simulink model "bldc_control_sim"  (R2021b)
settings: Solver=VariableStepAuto  StartTime=0.0  StopTime=30  RelTol=1e-3
InitFcn:
  | run bldc_control_params
values from neighbouring files (symbols this model uses):
  B = 2.63687521782e-06    [bldc_control_params.m]
  delay_Currents = 2    [bldc_control_params.m]
  enc_res = 16    [bldc_control_params.m]
  J = 7.06155183-06    (= 1.06155183)    [bldc_control_params.m]
  Ki_i = 3.7e3    (= 3700)    [bldc_control_params.m]
  Ki_speed = 0.1    [bldc_control_params.m]
  Kp_i = 2    [bldc_control_params.m]
  Kp_speed = 5    [bldc_control_params.m]
  poles = 14    [bldc_control_params.m]
  PositionOffset = 0.0    (= 0)    [bldc_control_params.m]
  T_pwm = 20000    [bldc_control_params.m]
  T_rated = 2    [bldc_control_params.m]
  Ts = 5.0e-5    (= 5e-05)    [bldc_control_params.m]
  Ts_inverter = 2.5e-5    (= 2.5e-05)    [bldc_control_params.m]
  Ts_motor = 2.5e-5    (= 2.5e-05)    [bldc_control_params.m]
  Ts_simulink = 2.5e-5    (= 2.5e-05)    [bldc_control_params.m]
  Ts_speed = 5.0e-4    (= 0.0005)    [bldc_control_params.m]
  V_dc = 15    [bldc_control_params.m]
libraries: mcbcontrolslib x19, mcbpositiondecoderlib x4, autolibpmsmexterior x1
settings Model: Creator=vasko  LastModifiedBy=vasko

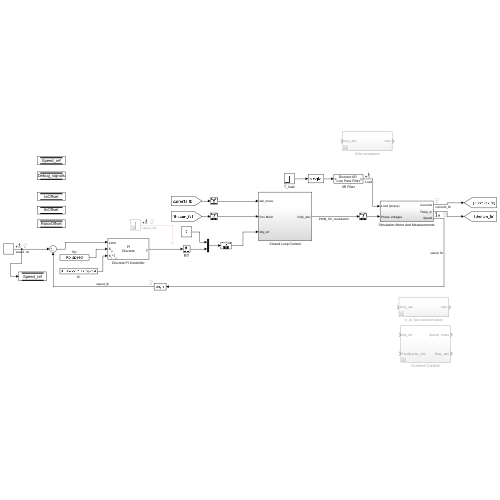
[thumbnail: Simulink's stored preview of the top-level diagram]
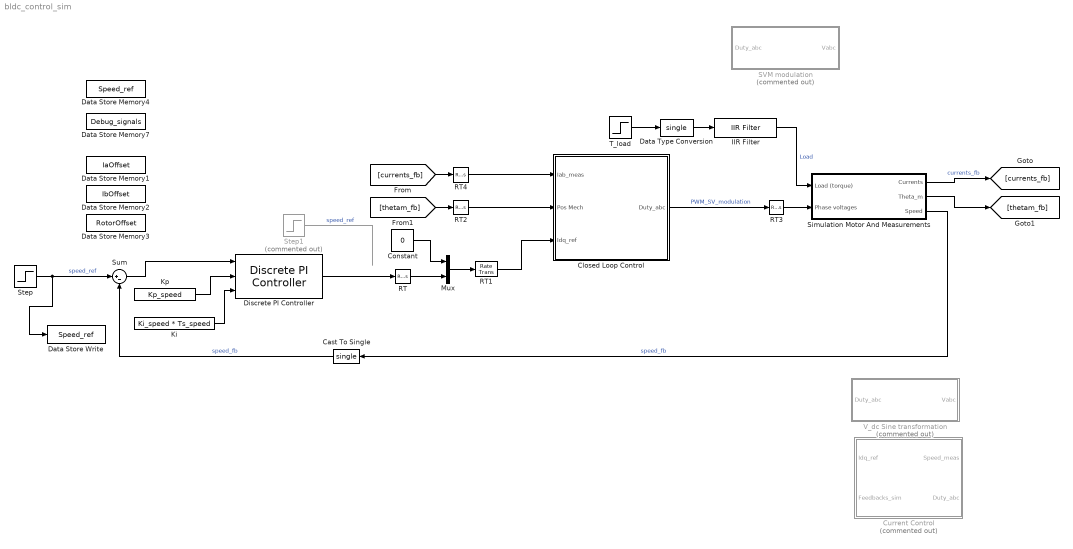
== system bldc_control_sim ==
  Cast To Single : DataTypeConversion  OutDataTypeStr=single
  Closed Loop Control : Subsystem
  Constant : Constant  Value=0  OutDataTypeStr=single
  Current Control : Subsystem  Commented=on
      settings: RTWSystemCode=Nonreusable function
  Data Store Memory1 : DataStoreMemory  DataStoreName=IaOffset  InitialValue=2064  ShowAdditionalParam=off  OutDataTypeStr=uint16
  Data Store Memory2 : DataStoreMemory  DataStoreName=IbOffset  InitialValue=2064  ShowAdditionalParam=off  OutDataTypeStr=uint16
  Data Store Memory3 : DataStoreMemory  DataStoreName=RotorOffset  InitialValue=2064  ShowAdditionalParam=off  OutDataTypeStr=uint16
  Data Store Memory4 : DataStoreMemory  DataStoreName=Speed_ref  ShowAdditionalParam=off  OutDataTypeStr=dataType
  Data Store Memory7 : DataStoreMemory  DataStoreName=Debug_signals  InitialValue=5  ShowAdditionalParam=off  OutDataTypeStr=uint16
  Data Store Write : DataStoreWrite  DataStoreName=Speed_ref  IndexOptions=Index vector (dialog)  Indices=1  OutputSizes=1
  Data Type Conversion : DataTypeConversion  OutDataTypeStr=single
  Discrete PI Controller : mcbcontrolslib/Discrete PI Controller
      settings: SourceProductBaseCode=MT
  IIR Filter : mcbcontrolslib/IIR Filter  VariantControl=Low Pass Filter  VariantSelect=Low-pass  Filter_constant=0.01  advancedSettings=off  Ts=50e-6  cutOff_freq=32.1525
      settings: SourceProductBaseCode=MT
  Ki : Constant  Value=Ki_speed * Ts_speed  OutDataTypeStr=dataType  SampleTime=-1
  Kp : Constant  Value=Kp_speed  OutDataTypeStr=dataType  SampleTime=-1
  Mux : Mux  Inputs=2
  RT : RateTransition  Deterministic=off  OutPortSampleTime=Ts_speed
  RT{1..4} (4 alike) : RateTransition  Deterministic=off
  SVM modulation : Subsystem  Commented=on
  Simulation Motor And Measurements : Subsystem
  Step : Step  After=2  OutDataTypeStr=single  SampleTime=Ts_simulink
  Step1 : Step  Commented=on  After=100  OutDataTypeStr=single  SampleTime=Ts_simulink
  Sum : Sum  Inputs=|+-
  T_load : Step  Time=1.5  After=0*T_rated  SampleTime=Ts_simulink
  V_dc Sine transformation : Subsystem  Commented=on
  wires:
  Simulation Motor And Measurements/1(Currents) -> [currents_fb]  "currents_fb"
  [currents_fb] -> RT4/1
  Step/1 -> Sum/1, Data Store Write/1  "speed_ref"
  RT/1 -> Mux/2
  Data Type Conversion/1 -> IIR Filter/1
  IIR Filter/1 -> Simulation Motor And Measurements/1(Load (torque))  "Load"
  Constant/1 -> Mux/1
  Mux/1 -> RT1/1
  T_load/1 -> Data Type Conversion/1
  Closed Loop Control/1(Duty_abc) -> RT3/1  "PWM_SV_modulation"
  RT2/1 -> Closed Loop Control/2(Pos Mech)
  RT4/1 -> Closed Loop Control/1(Iab_meas)
  RT1/1 -> Closed Loop Control/3(Idq_ref)
  RT3/1 -> Simulation Motor And Measurements/2(Phase voltages)
  [thetam_fb] -> RT2/1
  Simulation Motor And Measurements/2(Theta_m) -> [thetam_fb]
  Simulation Motor And Measurements/3(Speed) -> Cast To Single/1  "speed_fb"
  Sum/1 -> Discrete PI Controller/1
  Ki/1 -> Discrete PI Controller/3
  Kp/1 -> Discrete PI Controller/2
  Cast To Single/1 -> Sum/2  "speed_fb"
  Step1/1 -> ?  "speed_ref"
  Discrete PI Controller/1 -> RT/1

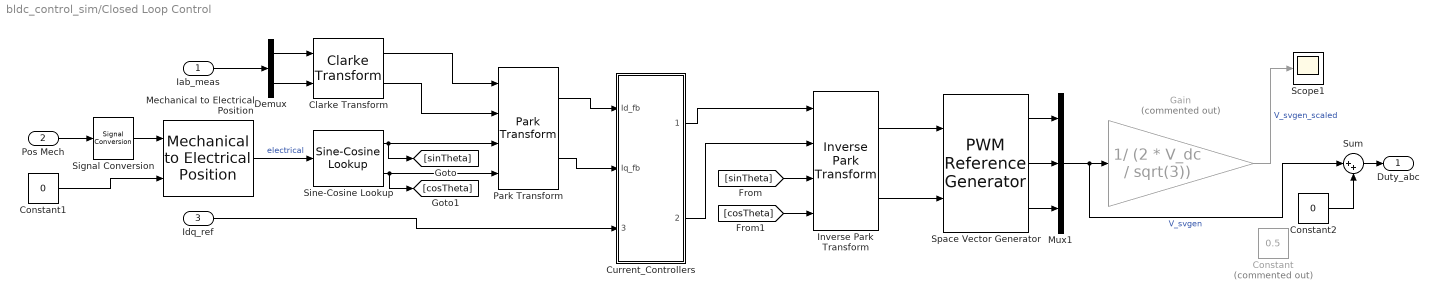
== system bldc_control_sim/Closed Loop Control ==
  Iab_meas : Inport
  Pos Mech : Inport  Port=2
  Idq_ref : Inport  Port=3
  Clarke Transform : mcbcontrolslib/Clarke Transform  VariantControl=Variant2
  Constant : Constant  Commented=on  Value=0.5  OutDataTypeStr=dataType  SampleTime=-1
  Constant1 : Constant  Value=0
  Constant2 : Constant  Value=0
  Current_Controllers : Subsystem
  Demux : Demux  Outputs=2
  Gain : Gain  Commented=on  Gain=1/ (2 * V_dc / sqrt(3))  RndMeth=Simplest  OutDataTypeStr=Inherit: Same as input
  Inverse Park Transform : mcbcontrolslib/Inverse Park Transform  AxisAlignment=D-axis
  Mechanical to Electrical Position : mcbpositiondecoderlib/Mechanical to Electrical Position  NrPP=poles  selectedRange=Radians  MechOfstInputType=Input port  mechOffsetIn=0  maxAngleIn=2*pi  InputDataType=dataType  VariantSelect=floating-point
      settings: SourceProductBaseCode=MT
  Mux1 : Mux  Inputs=3
  Park Transform : mcbcontrolslib/Park Transform  AxisAlignment=D-axis
      settings: SourceProductBaseCode=MT
  Scope1 : Scope
  Signal Conversion : SignalConversion  OverrideOpt=off
  Sine-Cosine Lookup : mcbcontrolslib/Sine-Cosine Lookup  AngleInput=Radians  N_points=1024
      settings: SourceProductBaseCode=MT
  Space Vector Generator : mcbcontrolslib/PWM Reference Generator  inSignal=Valphabeta  modType=SVM: space vector modulation
      settings: SourceProductBaseCode=MT
  Sum : Sum  Inputs=|++
  Duty_abc : Outport  VectorParamsAs1DForOutWhenUnconnected=off
  wires:
  Iab_meas/1 -> Demux/1
  Park Transform/2 -> Current_Controllers/2(Iq_fb)
  Park Transform/1 -> Current_Controllers/1(Id_fb)
  Sine-Cosine Lookup/2 -> Park Transform/4, [cosTheta]
  Clarke Transform/1 -> Park Transform/1
  Idq_ref/1 -> Current_Controllers/3(Idq_ref)
  Sine-Cosine Lookup/1 -> [sinTheta], Park Transform/3
  Clarke Transform/2 -> Park Transform/2
  [cosTheta] -> Inverse Park Transform/4
  Demux/2 -> Clarke Transform/2
  Demux/1 -> Clarke Transform/1
  [sinTheta] -> Inverse Park Transform/3
  Current_Controllers/1(Vd_ref) -> Inverse Park Transform/1
  Current_Controllers/2(Vq_ref) -> Inverse Park Transform/2
  Inverse Park Transform/2 -> Space Vector Generator/2
  Mux1/1 -> Sum/1, Gain/1  "V_svgen"
  Space Vector Generator/1 -> Mux1/1
  Gain/1 -> Scope1/1  "V_svgen_scaled"
  Inverse Park Transform/1 -> Space Vector Generator/1
  Space Vector Generator/2 -> Mux1/2
  Space Vector Generator/3 -> Mux1/3
  Sum/1 -> Duty_abc/1
  Pos Mech/1 -> Signal Conversion/1
  Mechanical to Electrical Position/1 -> Sine-Cosine Lookup/1  "electrical"
  Constant1/1 -> Mechanical to Electrical Position/2
  Constant2/1 -> Sum/2
  Signal Conversion/1 -> Mechanical to Electrical Position/1

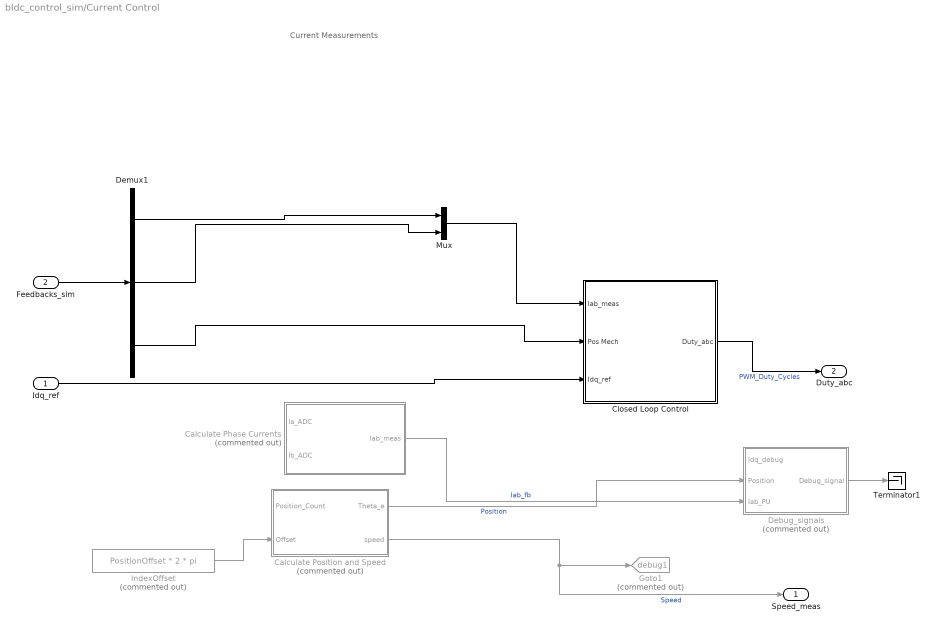
== system bldc_control_sim/Current Control ==
  note: Current Measurements
  Idq_ref : Inport
  Feedbacks_sim : Inport  Port=2
  " Calculate Position and Speed" : Subsystem  Commented=on
  Calculate Phase Currents : Subsystem  Commented=on
  Closed Loop Control : Subsystem
  Debug_signals : Subsystem  Commented=on
  Demux1 : Demux  Outputs=3
  Goto1 : Goto  Commented=on  GotoTag=debug1  TagVisibility=global
  IndexOffset : Constant  Commented=on  Value=PositionOffset * 2 * pi  OutDataTypeStr=dataType  SampleTime=-1
  Mux : Mux  Inputs=2
  Terminator1 : Terminator
  Speed_meas : Outport  InitialOutput=0  VectorParamsAs1DForOutWhenUnconnected=off
  Duty_abc : Outport  Port=2  VectorParamsAs1DForOutWhenUnconnected=off
  wires:
  " Calculate Position and Speed"/1(Theta_e) -> Debug_signals/2(Position)  "Position"
  " Calculate Position and Speed"/2(speed) -> Speed_meas/1, Goto1/1  "Speed"
  Calculate Phase Currents/1(Iab_meas) -> Debug_signals/3(Iab_PU)  "Iab_fb"
  Debug_signals/1(Debug_signal) -> Terminator1/1
  IndexOffset/1 -> " Calculate Position and Speed"/2(Offset)
  Idq_ref/1 -> Closed Loop Control/3(Idq_ref)
  Closed Loop Control/1(Duty_abc) -> Duty_abc/1  "PWM_Duty_Cycles"
  Feedbacks_sim/1 -> Demux1/1
  Demux1/1 -> Mux/1
  Demux1/2 -> Mux/2
  Demux1/3 -> Closed Loop Control/2(Pos Mech)
  Mux/1 -> Closed Loop Control/1(Iab_meas)

== system bldc_control_sim/SVM modulation ==
  Duty_abc : Inport
  Average_Value_Inverter : Subsystem
  Constant2 : Constant  Value=V_dc  OutDataTypeStr=single  SampleTime=-1
  Data Type Conversion1 : DataTypeConversion  OutDataTypeStr=single  RndMeth=Simplest
  Demux : Demux  Outputs=3
  Inverter_delay : DiscreteTransferFcn  Numerator=[1-exp(-Ts_inverter/(T_pwm/2))]  Denominator=[1 -exp(-Ts_inverter/(T_pwm/2))]  RndMeth=Simplest
  Mux : Mux  Inputs=3
  Rate Transition3 : RateTransition  Integrity=off  OutPortSampleTime=Ts_inverter
  Vabc : Outport  VectorParamsAs1DForOutWhenUnconnected=off
  wires:
  Average_Value_Inverter/2(Vb) -> Mux/2
  Mux/1 -> Inverter_delay/1
  Constant2/1 -> Average_Value_Inverter/4(Vdc)
  Average_Value_Inverter/3(Vc) -> Mux/3
  Average_Value_Inverter/1(Va) -> Mux/1
  Demux/1 -> Average_Value_Inverter/1(Vao)
  Demux/3 -> Average_Value_Inverter/3(Vco)
  Demux/2 -> Average_Value_Inverter/2(Vbo)
  Data Type Conversion1/1 -> Rate Transition3/1
  Rate Transition3/1 -> Demux/1
  Inverter_delay/1 -> Vabc/1
  Duty_abc/1 -> Data Type Conversion1/1

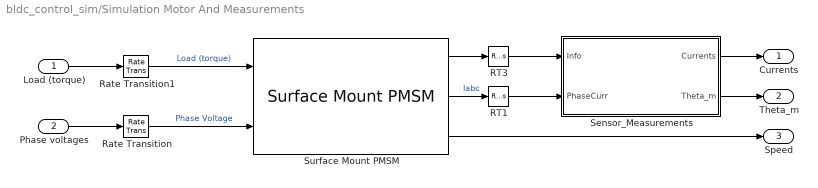
== system bldc_control_sim/Simulation Motor And Measurements ==
  Load (torque) : Inport
  Phase voltages : Inport  Port=2
  RT1 : RateTransition  Deterministic=off  OutPortSampleTime=Ts_simulink
  RT3 : RateTransition  Deterministic=off  OutPortSampleTime=Ts_simulink
  Rate Transition : RateTransition  Integrity=off  OutPortSampleTime=Ts_motor
  Rate Transition1 : RateTransition  Integrity=off  OutPortSampleTime=Ts_motor
  Sensor_Measurements : Subsystem
  Surface Mount PMSM : autolibpmsmexterior/Surface Mount PMSM  port_config=Torque  sim_type=Discrete  Ts=Ts_motor  P=poles  Rs=Rs  Ldq_=Ld  KConstText=Permanent flux linkage constant (lambda_pm):  lambda_pm=FluxPM  Ke=159.9771  Kt=1.323  mechanical=[J, B, 0]  idq0=[0 0]  theta_init=0  omega_init=0  KConst=FluxPM  lambda_pm_calc=FluxPM  RefBlkName='autolibpmsmexterior/Surface Mount PMSM'  aMode=5  Ldq="[0.00105     0.00105]"
      settings: SourceProductBaseCode=PW,DR,MT,UV,VE
  Currents : Outport  VectorParamsAs1DForOutWhenUnconnected=off
  Theta_m : Outport  Port=2  VectorParamsAs1DForOutWhenUnconnected=off
  Speed : Outport  Port=3  VectorParamsAs1DForOutWhenUnconnected=off
  wires:
  Rate Transition1/1 -> Surface Mount PMSM/1  "Load (torque)"
  Surface Mount PMSM/2 -> RT1/1  "Iabc"
  Surface Mount PMSM/3 -> Speed/1
  Rate Transition/1 -> Surface Mount PMSM/2  "Phase Voltage"
  RT1/1 -> Sensor_Measurements/2(PhaseCurr)
  Phase voltages/1 -> Rate Transition/1
  RT3/1 -> Sensor_Measurements/1(Info)
  Surface Mount PMSM/1 -> RT3/1
  Load (torque)/1 -> Rate Transition1/1
  Sensor_Measurements/1(Currents) -> Currents/1
  Sensor_Measurements/2(Theta_m) -> Theta_m/1

== system bldc_control_sim/V_dc Sine transformation ==
  Duty_abc : Inport
  Average_Value_Inverter : Subsystem
  Constant2 : Constant  Value=V_dc  OutDataTypeStr=single  SampleTime=-1
  Data Type Conversion1 : DataTypeConversion  OutDataTypeStr=single  RndMeth=Simplest
  Demux : Demux  Outputs=3
  Mux : Mux  Inputs=3
  Rate Transition3 : RateTransition  Integrity=off  OutPortSampleTime=Ts_inverter
  Vabc : Outport  VectorParamsAs1DForOutWhenUnconnected=off
  wires:
  Average_Value_Inverter/2(Vb) -> Mux/2
  Constant2/1 -> Average_Value_Inverter/4(Vdc)
  Average_Value_Inverter/3(Vc) -> Mux/3
  Average_Value_Inverter/1(Va) -> Mux/1
  Demux/1 -> Average_Value_Inverter/1(Vao)
  Demux/3 -> Average_Value_Inverter/3(Vco)
  Demux/2 -> Average_Value_Inverter/2(Vbo)
  Data Type Conversion1/1 -> Rate Transition3/1
  Rate Transition3/1 -> Demux/1
  Mux/1 -> Vabc/1  "V_inv_abc"
  Duty_abc/1 -> Data Type Conversion1/1

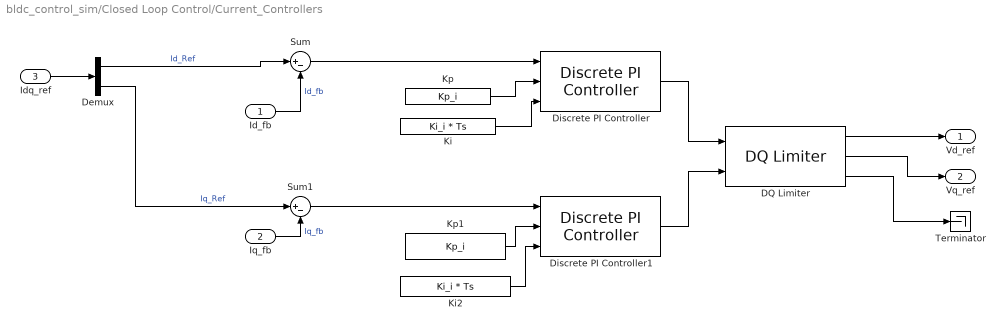
== system bldc_control_sim/Closed Loop Control/Current_Controllers ==
  Id_fb : Inport
  Iq_fb : Inport  Port=2
  Idq_ref : Inport  Port=3
  DQ Limiter : mcbcontrolslib/DQ Limiter  Vmax=Idq_lim
      settings: SourceProductBaseCode=MT
  Demux : Demux  Outputs=2
  Discrete PI Controller : mcbcontrolslib/Discrete PI Controller
      settings: SourceProductBaseCode=MT
  Discrete PI Controller1 : mcbcontrolslib/Discrete PI Controller
      settings: SourceProductBaseCode=MT
  Ki : Constant  Value=Ki_i * Ts  OutDataTypeStr=dataType  SampleTime=-1
  Ki2 : Constant  Value=Ki_i * Ts  OutDataTypeStr=dataType  SampleTime=-1
  Kp : Constant  Value=Kp_i  OutDataTypeStr=dataType  SampleTime=-1
  Kp1 : Constant  Value=Kp_i  OutDataTypeStr=dataType  SampleTime=-1
  Sum : Sum  Inputs=|+-  OutDataTypeStr=Inherit: Same as first input
  Sum1 : Sum  Inputs=|+-  OutDataTypeStr=Inherit: Same as first input
  Terminator : Terminator
  Vd_ref : Outport  VectorParamsAs1DForOutWhenUnconnected=off
  Vq_ref : Outport  Port=2  VectorParamsAs1DForOutWhenUnconnected=off
  wires:
  Iq_fb/1 -> Sum1/2  "Iq_fb"
  Id_fb/1 -> Sum/2  "Id_fb"
  Demux/1 -> Sum/1  "Id_Ref"
  Demux/2 -> Sum1/1  "Iq_Ref"
  Idq_ref/1 -> Demux/1
  DQ Limiter/2 -> Vq_ref/1
  DQ Limiter/1 -> Vd_ref/1
  DQ Limiter/3 -> Terminator/1
  Ki/1 -> Discrete PI Controller/3
  Sum/1 -> Discrete PI Controller/1
  Kp/1 -> Discrete PI Controller/2
  Sum1/1 -> Discrete PI Controller1/1
  Ki2/1 -> Discrete PI Controller1/3
  Kp1/1 -> Discrete PI Controller1/2
  Discrete PI Controller/1 -> DQ Limiter/1
  Discrete PI Controller1/1 -> DQ Limiter/2

== system bldc_control_sim/Current Control/ Calculate Position and Speed ==
  Position_Count : Inport
  Offset : Inport  Port=2
  Cast To Single : DataTypeConversion  OutDataTypeStr=single
  Gain : Gain  Gain=2*pi/(2^enc_res)
  IIR Filter : mcbcontrolslib/IIR Filter  VariantControl=Low Pass Filter  VariantSelect=Low-pass  Filter_constant=0.01  advancedSettings=off  Ts=50e-6  cutOff_freq=32.1525
      settings: SourceProductBaseCode=MT
  Mechanical to Electrical Position : mcbpositiondecoderlib/Mechanical to Electrical Position  NrPP=poles  selectedRange=Radians  MechOfstInputType=Input port  mechOffsetIn=0  maxAngleIn=2*pi  InputDataType=dataType  VariantSelect=floating-point
      settings: SourceProductBaseCode=MT
  Speed Measurement : mcbpositiondecoderlib/Speed Measurement  PositionUnit=Radians  PositionScalingDatatype=uint32  SpeedCalculationMode=Time interval for speed calculation  SampleTimeAsync=Ts  MaximumApplicationSpeed=6000  SpeedResolution=5e-6  DelayLength=20  MaximumMeasurableSpeed=29999  MeasurableSpeedResolution=1.397e-05  SpeedUnit=Radians/Sec  PerUnitSpeed=PU_System.N_base  SpeedDataType=dataType
      settings: SourceProductBaseCode=MT
  Theta_e : Outport  VectorParamsAs1DForOutWhenUnconnected=off
  speed : Outport  Port=2  VectorParamsAs1DForOutWhenUnconnected=off
  wires:
  Speed Measurement/1 -> IIR Filter/1
  Mechanical to Electrical Position/1 -> Theta_e/1
  Position_Count/1 -> Gain/1
  Offset/1 -> Mechanical to Electrical Position/2
  IIR Filter/1 -> speed/1
  Gain/1 -> Cast To Single/1
  Cast To Single/1 -> Speed Measurement/1, Mechanical to Electrical Position/1  "angle"

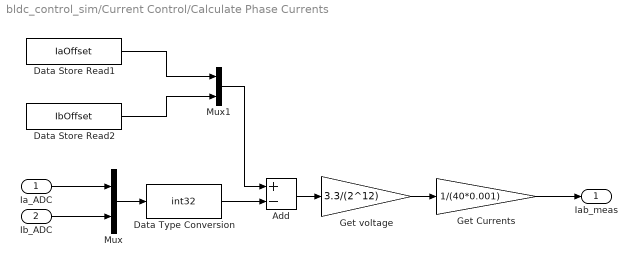
== system bldc_control_sim/Current Control/Calculate Phase Currents ==
  Ia_ADC : Inport
  Ib_ADC : Inport  Port=2
  Add : Sum  Inputs=+-
  Data Store Read1 : DataStoreRead  DataStoreName=IaOffset  IndexOptions=Index vector (dialog)  Indices=1  OutputSizes=1
  Data Store Read2 : DataStoreRead  DataStoreName=IbOffset  IndexOptions=Index vector (dialog)  Indices=1  OutputSizes=1
  Data Type Conversion : DataTypeConversion  OutDataTypeStr=int32  ConvertRealWorld=Stored Integer (SI)  RndMeth=Simplest
  Get Currents : Gain  Gain=1/(40*0.001)  OutDataTypeStr=dataType  RndMeth=Simplest
  Get voltage : Gain  Gain=3.3/(2^12)
  Mux : Mux  Inputs=2
  Mux1 : Mux  Inputs=2
  Iab_meas : Outport  VectorParamsAs1DForOutWhenUnconnected=off
  wires:
  Data Type Conversion/1 -> Add/2
  Ia_ADC/1 -> Mux/1
  Ib_ADC/1 -> Mux/2
  Mux/1 -> Data Type Conversion/1
  Data Store Read1/1 -> Mux1/1
  Data Store Read2/1 -> Mux1/2
  Mux1/1 -> Add/1
  Get Currents/1 -> Iab_meas/1
  Add/1 -> Get voltage/1
  Get voltage/1 -> Get Currents/1

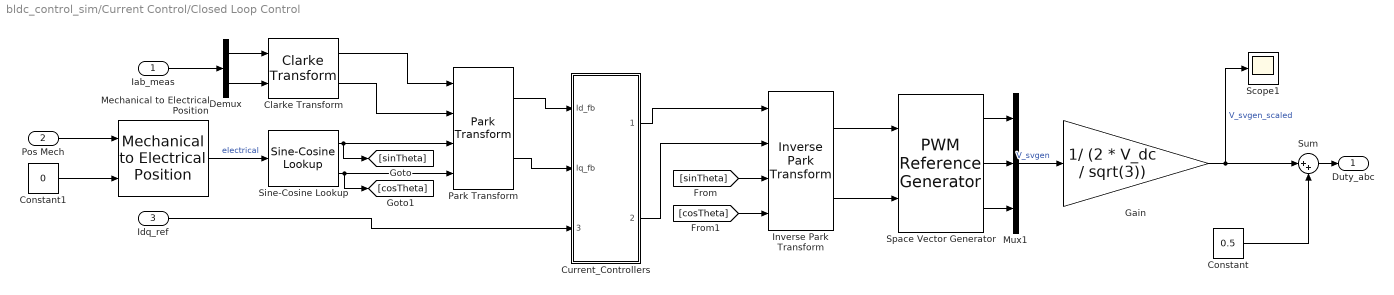
== system bldc_control_sim/Current Control/Closed Loop Control ==
  Iab_meas : Inport
  Pos Mech : Inport  Port=2
  Idq_ref : Inport  Port=3
  Clarke Transform : mcbcontrolslib/Clarke Transform  VariantControl=Variant2
  Constant : Constant  Value=0.5  OutDataTypeStr=dataType  SampleTime=-1
  Constant1 : Constant  Value=0
  Current_Controllers : Subsystem
  Demux : Demux  Outputs=2
  Gain : Gain  Gain=1/ (2 * V_dc / sqrt(3))  RndMeth=Simplest  OutDataTypeStr=Inherit: Same as input
  Inverse Park Transform : mcbcontrolslib/Inverse Park Transform  AxisAlignment=D-axis
  Mechanical to Electrical Position : mcbpositiondecoderlib/Mechanical to Electrical Position  NrPP=poles  selectedRange=Radians  MechOfstInputType=Input port  mechOffsetIn=0  maxAngleIn=2*pi  InputDataType=dataType  VariantSelect=floating-point
      settings: SourceProductBaseCode=MT
  Mux1 : Mux  Inputs=3
  Park Transform : mcbcontrolslib/Park Transform  AxisAlignment=D-axis
      settings: SourceProductBaseCode=MT
  Scope1 : Scope
  Sine-Cosine Lookup : mcbcontrolslib/Sine-Cosine Lookup  AngleInput=Radians  N_points=1024
      settings: SourceProductBaseCode=MT
  Space Vector Generator : mcbcontrolslib/PWM Reference Generator  inSignal=Valphabeta  modType=SVM: space vector modulation
      settings: SourceProductBaseCode=MT
  Sum : Sum  Inputs=|++
  Duty_abc : Outport  VectorParamsAs1DForOutWhenUnconnected=off
  wires:
  Iab_meas/1 -> Demux/1
  Park Transform/2 -> Current_Controllers/2(Iq_fb)
  Park Transform/1 -> Current_Controllers/1(Id_fb)
  Sine-Cosine Lookup/2 -> Park Transform/4, [cosTheta]
  Clarke Transform/1 -> Park Transform/1
  Idq_ref/1 -> Current_Controllers/3(Idq_ref)
  Sine-Cosine Lookup/1 -> [sinTheta], Park Transform/3
  Clarke Transform/2 -> Park Transform/2
  [cosTheta] -> Inverse Park Transform/4
  Demux/2 -> Clarke Transform/2
  Demux/1 -> Clarke Transform/1
  [sinTheta] -> Inverse Park Transform/3
  Current_Controllers/1(Vd_ref) -> Inverse Park Transform/1
  Current_Controllers/2(Vq_ref) -> Inverse Park Transform/2
  Inverse Park Transform/2 -> Space Vector Generator/2
  Constant/1 -> Sum/2
  Mux1/1 -> Gain/1  "V_svgen"
  Space Vector Generator/1 -> Mux1/1
  Gain/1 -> Scope1/1, Sum/1  "V_svgen_scaled"
  Inverse Park Transform/1 -> Space Vector Generator/1
  Space Vector Generator/2 -> Mux1/2
  Space Vector Generator/3 -> Mux1/3
  Sum/1 -> Duty_abc/1
  Pos Mech/1 -> Mechanical to Electrical Position/1
  Mechanical to Electrical Position/1 -> Sine-Cosine Lookup/1  "electrical"
  Constant1/1 -> Mechanical to Electrical Position/2

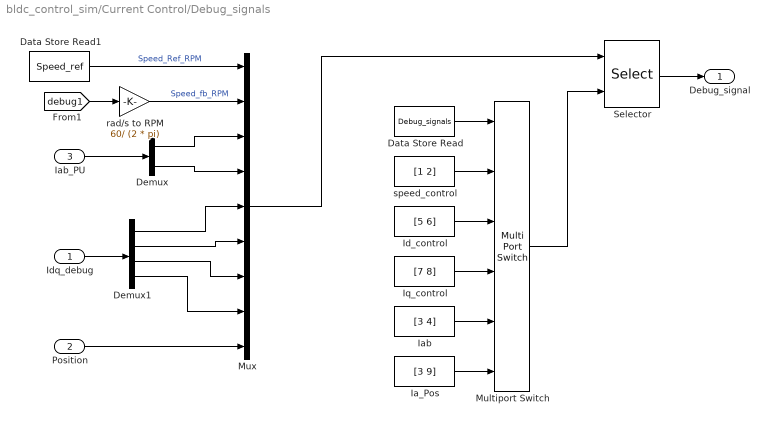
== system bldc_control_sim/Current Control/Debug_signals ==
  Idq_debug : Inport
  Position : Inport  Port=2
  Iab_PU : Inport  Port=3
  Data Store Read : DataStoreRead  DataStoreName=Debug_signals  IndexOptions=Index vector (dialog)  Indices=1  OutputSizes=1
  Data Store Read1 : DataStoreRead  DataStoreName=Speed_ref  IndexOptions=Index vector (dialog)  Indices=1  OutputSizes=1
  Demux : Demux  Outputs=2
  Demux1 : Demux
  Ia_Pos : Constant  Value=[3 9]  OutDataTypeStr=uint16  SampleTime=-1
  Iab : Constant  Value=[3 4]  OutDataTypeStr=uint16  SampleTime=-1
  Id_control : Constant  Value=[5 6]  OutDataTypeStr=uint16  SampleTime=-1
  Iq_control : Constant  Value=[7 8]  OutDataTypeStr=uint16  SampleTime=-1
  Multiport Switch : MultiPortSwitch  Inputs=5  DiagnosticForDefault=Warning  OutDataTypeStr=uint16  RndMeth=Simplest
  Mux : Mux  Inputs=9
  Selector : Selector  InputPortWidth=9  IndexOptions=Index vector (port)  Indices=[1 3]  OutputSizes=1
  rad/s to RPM : Gain  Gain=60/ (2 * pi)  RndMeth=Simplest  OutDataTypeStr=Inherit: Same as input
  speed_control : Constant  Value=[1 2]  OutDataTypeStr=uint16  SampleTime=-1
  Debug_signal : Outport
  wires:
  speed_control/1 -> Multiport Switch/2
  Id_control/1 -> Multiport Switch/3
  Iq_control/1 -> Multiport Switch/4
  Iab/1 -> Multiport Switch/5
  Ia_Pos/1 -> Multiport Switch/6
  Multiport Switch/1 -> Selector/2
  Data Store Read/1 -> Multiport Switch/1
  Selector/1 -> Debug_signal/1
  Iab_PU/1 -> Demux/1
  Demux/1 -> Mux/3
  Demux/2 -> Mux/4
  Demux1/1 -> Mux/5
  Demux1/2 -> Mux/6
  Demux1/3 -> Mux/7
  Demux1/4 -> Mux/8
  Idq_debug/1 -> Demux1/1
  Mux/1 -> Selector/1
  Position/1 -> Mux/9
  [debug1] -> rad/s to RPM/1
  Data Store Read1/1 -> Mux/1  "Speed_Ref_RPM"
  rad/s to RPM/1 -> Mux/2  "Speed_fb_RPM"

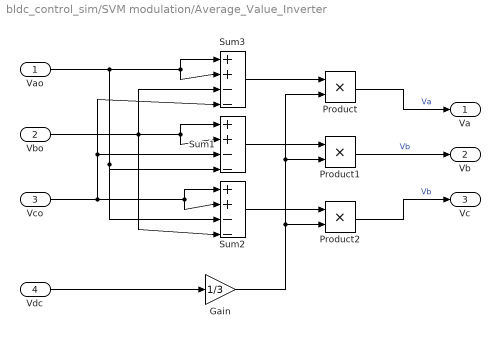
== system bldc_control_sim/SVM modulation/Average_Value_Inverter ==
  Vao : Inport
  Vbo : Inport  Port=2
  Vco : Inport  Port=3
  Vdc : Inport  Port=4
  Gain : Gain  Gain=1/3  RndMeth=Simplest  OutDataTypeStr=Inherit: Same as input
  Product : Product  RndMeth=Simplest  OutDataTypeStr=Inherit: Same as first input
  Product1 : Product  RndMeth=Simplest  OutDataTypeStr=Inherit: Same as first input
  Product2 : Product  RndMeth=Simplest  OutDataTypeStr=Inherit: Same as first input
  Sum1 : Sum  Inputs=|++--  RndMeth=Simplest  OutDataTypeStr=Inherit: Same as first input
  Sum2 : Sum  Inputs=|++--  RndMeth=Simplest  OutDataTypeStr=Inherit: Same as first input
  Sum3 : Sum  Inputs=|++--  RndMeth=Simplest  OutDataTypeStr=Inherit: Same as first input
  Va : Outport  VectorParamsAs1DForOutWhenUnconnected=off
  Vb : Outport  Port=2  VectorParamsAs1DForOutWhenUnconnected=off
  Vc : Outport  Port=3  VectorParamsAs1DForOutWhenUnconnected=off
  wires:
  Product1/1 -> Vb/1  "Vb"
  Gain/1 -> Product/2, Product1/2, Product2/2
  Sum2/1 -> Product2/1
  Vao/1 -> Sum3/1, Sum3/2, Sum1/4, Sum2/3
  Product2/1 -> Vc/1  "Vb"
  Sum1/1 -> Product1/1
  Vdc/1 -> Gain/1
  Sum3/1 -> Product/1
  Product/1 -> Va/1  "Va"
  Vco/1 -> Sum3/4, Sum1/3, Sum2/2, Sum2/1
  Vbo/1 -> Sum1/1, Sum1/2, Sum3/3, Sum2/4

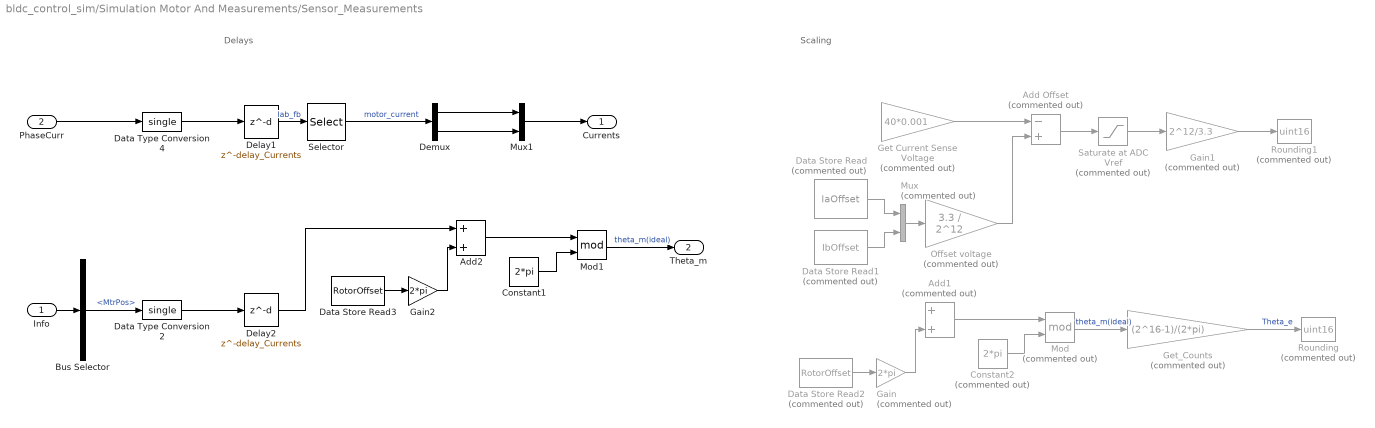
== system bldc_control_sim/Simulation Motor And Measurements/Sensor_Measurements ==
  note: Scaling
  note: Delays
  Info : Inport
  PhaseCurr : Inport  Port=2
  Add Offset : Sum  Commented=on  Inputs=-+  RndMeth=Simplest
  Add1 : Sum  Commented=on  RndMeth=Simplest
  Add2 : Sum  RndMeth=Simplest
  Bus Selector : BusSelector  OutputSignals=MtrPos
  Constant1 : Constant  Value=2*pi  OutDataTypeStr=single  SampleTime=-1
  Constant2 : Constant  Commented=on  Value=2*pi  OutDataTypeStr=single  SampleTime=-1
  Data Store Read : DataStoreRead  Commented=on  DataStoreName=IaOffset  IndexOptions=Index vector (dialog)  Indices=1  OutputSizes=1
  Data Store Read1 : DataStoreRead  Commented=on  DataStoreName=IbOffset  IndexOptions=Index vector (dialog)  Indices=1  OutputSizes=1
  Data Store Read2 : DataStoreRead  Commented=on  DataStoreName=RotorOffset  IndexOptions=Index vector (dialog)  Indices=1  OutputSizes=1
  Data Store Read3 : DataStoreRead  DataStoreName=RotorOffset  IndexOptions=Index vector (dialog)  Indices=1  OutputSizes=1
  Data Type Conversion2 : DataTypeConversion  OutDataTypeStr=single  RndMeth=Simplest
  Data Type Conversion4 : DataTypeConversion  OutDataTypeStr=single  RndMeth=Simplest
  Delay1 : Delay  DelayLength=delay_Currents
  Delay2 : Delay  DelayLength=delay_Currents
  Demux : Demux  Outputs=2
  Gain : Gain  Commented=on  Gain=2*pi
  Gain1 : Gain  Commented=on  Gain=2^12/3.3
  Gain2 : Gain  Gain=2*pi
  Get Current Sense Voltage : Gain  Commented=on  Gain=40*0.001  RndMeth=Simplest  OutDataTypeStr=Inherit: Same as input
  Get_Counts : Gain  Commented=on  Gain=(2^16-1)/(2*pi)  OutDataTypeStr=uint16  RndMeth=Simplest
  Mod : Math  Commented=on  Operator=mod  SaturateOnIntegerOverflow=on
  Mod1 : Math  Operator=mod  SaturateOnIntegerOverflow=on
  Mux : Mux  Commented=on  Inputs=2
  Mux1 : Mux  Inputs=2
  Offset voltage : Gain  Commented=on  Gain=3.3 / 2^12  RndMeth=Simplest
  Rounding : DataTypeConversion  Commented=on  OutDataTypeStr=uint16  RndMeth=Simplest
  Rounding1 : DataTypeConversion  Commented=on  OutDataTypeStr=uint16  RndMeth=Simplest
  Saturate at ADC Vref : Saturate  Commented=on  UpperLimit=3.3  LowerLimit=0
  Selector : Selector  InputPortWidth=3  IndexOptions=Index vector (dialog)  Indices=[1 2]  OutputSizes=1
  Currents : Outport  VectorParamsAs1DForOutWhenUnconnected=off
  Theta_m : Outport  Port=2  VectorParamsAs1DForOutWhenUnconnected=off
  wires:
  Delay1/1 -> Selector/1  "Iab_fb"
  Data Type Conversion4/1 -> Delay1/1
  PhaseCurr/1 -> Data Type Conversion4/1
  Info/1 -> Bus Selector/1
  Bus Selector/1 -> Data Type Conversion2/1  "<MtrPos>"
  Data Type Conversion2/1 -> Delay2/1
  Data Store Read2/1 -> Gain/1
  Add1/1 -> Mod/1
  Get_Counts/1 -> Rounding/1  "Theta_e"
  Mod/1 -> Get_Counts/1  "theta_m(ideal)"
  Mux/1 -> Offset voltage/1
  Get Current Sense Voltage/1 -> Add Offset/1
  Saturate at ADC Vref/1 -> Gain1/1
  Add Offset/1 -> Saturate at ADC Vref/1
  Offset voltage/1 -> Add Offset/2
  Gain1/1 -> Rounding1/1
  Data Store Read1/1 -> Mux/2
  Data Store Read/1 -> Mux/1
  Constant2/1 -> Mod/2
  Gain/1 -> Add1/2
  Selector/1 -> Demux/1  "motor_current"
  Gain2/1 -> Add2/2
  Constant1/1 -> Mod1/2
  Add2/1 -> Mod1/1
  Data Store Read3/1 -> Gain2/1
  Mod1/1 -> Theta_m/1  "theta_m(ideal)"
  Delay2/1 -> Add2/1
  Demux/1 -> Mux1/1
  Demux/2 -> Mux1/2
  Mux1/1 -> Currents/1

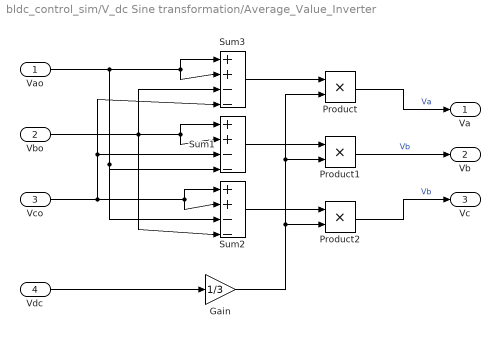
== system bldc_control_sim/V_dc Sine transformation/Average_Value_Inverter ==
  Vao : Inport
  Vbo : Inport  Port=2
  Vco : Inport  Port=3
  Vdc : Inport  Port=4
  Gain : Gain  Gain=1/3  RndMeth=Simplest  OutDataTypeStr=Inherit: Same as input
  Product : Product  RndMeth=Simplest  OutDataTypeStr=Inherit: Same as first input
  Product1 : Product  RndMeth=Simplest  OutDataTypeStr=Inherit: Same as first input
  Product2 : Product  RndMeth=Simplest  OutDataTypeStr=Inherit: Same as first input
  Sum1 : Sum  Inputs=|++--  RndMeth=Simplest  OutDataTypeStr=Inherit: Same as first input
  Sum2 : Sum  Inputs=|++--  RndMeth=Simplest  OutDataTypeStr=Inherit: Same as first input
  Sum3 : Sum  Inputs=|++--  RndMeth=Simplest  OutDataTypeStr=Inherit: Same as first input
  Va : Outport  VectorParamsAs1DForOutWhenUnconnected=off
  Vb : Outport  Port=2  VectorParamsAs1DForOutWhenUnconnected=off
  Vc : Outport  Port=3  VectorParamsAs1DForOutWhenUnconnected=off
  wires:
  Product1/1 -> Vb/1  "Vb"
  Gain/1 -> Product/2, Product1/2, Product2/2
  Sum2/1 -> Product2/1
  Vao/1 -> Sum3/1, Sum3/2, Sum1/4, Sum2/3
  Product2/1 -> Vc/1  "Vb"
  Sum1/1 -> Product1/1
  Vdc/1 -> Gain/1
  Sum3/1 -> Product/1
  Product/1 -> Va/1  "Va"
  Vco/1 -> Sum3/4, Sum1/3, Sum2/2, Sum2/1
  Vbo/1 -> Sum1/1, Sum1/2, Sum3/3, Sum2/4

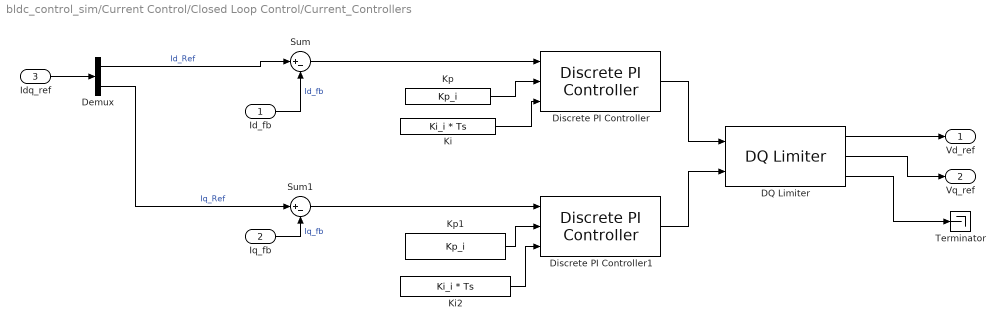
== system bldc_control_sim/Current Control/Closed Loop Control/Current_Controllers ==
  Id_fb : Inport
  Iq_fb : Inport  Port=2
  Idq_ref : Inport  Port=3
  DQ Limiter : mcbcontrolslib/DQ Limiter  Vmax=Idq_lim
      settings: SourceProductBaseCode=MT
  Demux : Demux  Outputs=2
  Discrete PI Controller : mcbcontrolslib/Discrete PI Controller
      settings: SourceProductBaseCode=MT
  Discrete PI Controller1 : mcbcontrolslib/Discrete PI Controller
      settings: SourceProductBaseCode=MT
  Ki : Constant  Value=Ki_i * Ts  OutDataTypeStr=dataType  SampleTime=-1
  Ki2 : Constant  Value=Ki_i * Ts  OutDataTypeStr=dataType  SampleTime=-1
  Kp : Constant  Value=Kp_i  OutDataTypeStr=dataType  SampleTime=-1
  Kp1 : Constant  Value=Kp_i  OutDataTypeStr=dataType  SampleTime=-1
  Sum : Sum  Inputs=|+-  OutDataTypeStr=Inherit: Same as first input
  Sum1 : Sum  Inputs=|+-  OutDataTypeStr=Inherit: Same as first input
  Terminator : Terminator
  Vd_ref : Outport  VectorParamsAs1DForOutWhenUnconnected=off
  Vq_ref : Outport  Port=2  VectorParamsAs1DForOutWhenUnconnected=off
  wires:
  Iq_fb/1 -> Sum1/2  "Iq_fb"
  Id_fb/1 -> Sum/2  "Id_fb"
  Demux/1 -> Sum/1  "Id_Ref"
  Demux/2 -> Sum1/1  "Iq_Ref"
  Idq_ref/1 -> Demux/1
  DQ Limiter/2 -> Vq_ref/1
  DQ Limiter/1 -> Vd_ref/1
  DQ Limiter/3 -> Terminator/1
  Ki/1 -> Discrete PI Controller/3
  Sum/1 -> Discrete PI Controller/1
  Kp/1 -> Discrete PI Controller/2
  Sum1/1 -> Discrete PI Controller1/1
  Ki2/1 -> Discrete PI Controller1/3
  Kp1/1 -> Discrete PI Controller1/2
  Discrete PI Controller/1 -> DQ Limiter/1
  Discrete PI Controller1/1 -> DQ Limiter/2
